simulink model "Model"  (R2024a)
settings: Solver=FixedStepDiscrete  StartTime=0.0  StopTime=inf  FixedStep=0.001  RelTol=1e-3
model workspace (MATLAB code in the model file):
  | Amplitude = 0.35/2;
settings Model: Creator=Are-Laptop  LastModifiedBy=Are-Laptop

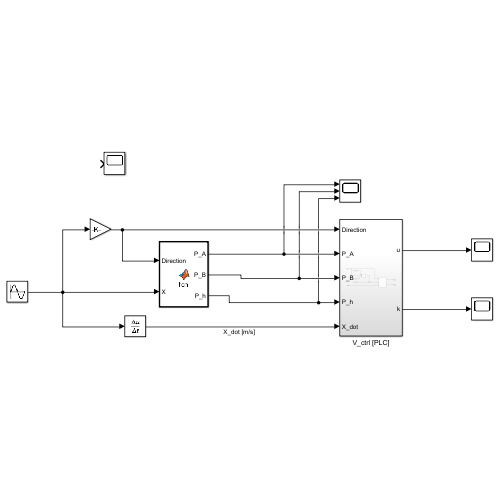
[thumbnail: Simulink's stored preview of the top-level diagram]
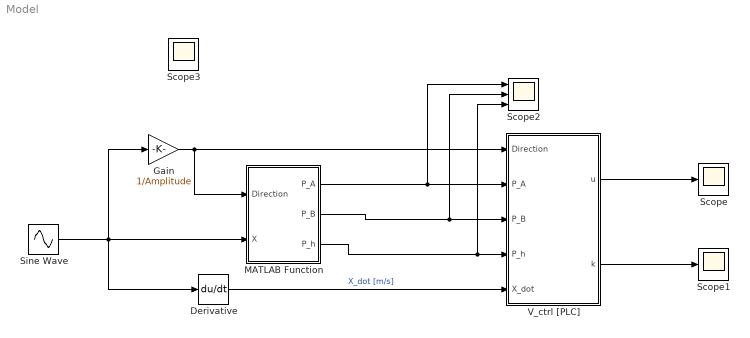
== system Model ==
  Derivative : Derivative
  Gain : Gain  Gain=1/Amplitude
  MATLAB Function : MATLAB Function  TreatAsAtomicUnit=on
  Scope : Scope
  Scope1 : Scope
  Scope2 : Scope  NumInputPorts=3
  Scope3 : Scope
  Sine Wave : Sin  Amplitude=Amplitude  Frequency=1/10  SampleTime=0
  V_ctrl [PLC] : Subsystem
  wires:
  MATLAB Function/2(P_B) -> Scope2/2, V_ctrl [PLC]/3(P_B)
  MATLAB Function/1(P_A) -> Scope2/1, V_ctrl [PLC]/2(P_A)
  MATLAB Function/3(P_h) -> Scope2/3, V_ctrl [PLC]/4(P_h)
  Derivative/1 -> V_ctrl [PLC]/5(X_dot)  "X_dot [m/s]"
  Gain/1 -> MATLAB Function/1(Direction), V_ctrl [PLC]/1(Direction)
  V_ctrl [PLC]/1(u) -> Scope/1
  V_ctrl [PLC]/2(k) -> Scope1/1
  Sine Wave/1 -> Derivative/1, Gain/1, MATLAB Function/2(X)

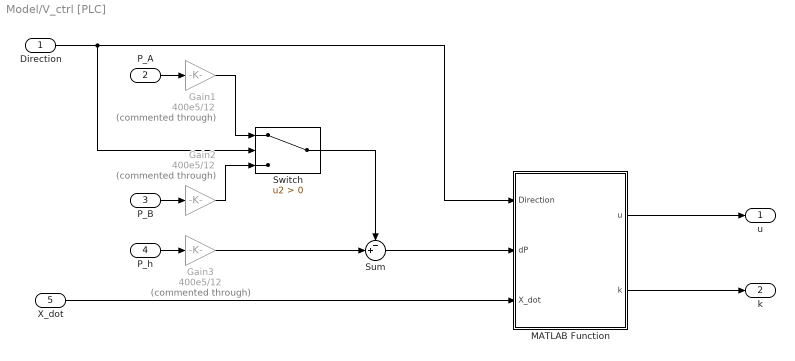
== system Model/V_ctrl [PLC] ==
  Direction : Inport
  P_A : Inport  Port=2
  P_B : Inport  Port=3
  P_h : Inport  Port=4
  X_dot : Inport  Port=5
  Gain1 : Gain  Commented=through  Gain=400e5/12
  Gain2 : Gain  Commented=through  Gain=400e5/12
  Gain3 : Gain  Commented=through  Gain=400e5/12
  MATLAB Function : MATLAB Function  TreatAsAtomicUnit=on
  Sum : Sum  Inputs=-+|
  Switch : Switch  Criteria=u2 > Threshold  SaturateOnIntegerOverflow=off  InputSameDT=off
  u : Outport
  k : Outport  Port=2
  wires:
  P_A/1 -> Gain1/1
  P_B/1 -> Gain2/1
  Direction/1 -> Switch/2, MATLAB Function/1(Direction)
  Sum/1 -> MATLAB Function/2(dP)
  P_h/1 -> Gain3/1
  Switch/1 -> Sum/1
  MATLAB Function/1(u) -> u/1
  Gain2/1 -> Switch/3
  Gain1/1 -> Switch/1
  Gain3/1 -> Sum/2
  X_dot/1 -> MATLAB Function/3(X_dot)
  MATLAB Function/2(k) -> k/1

== matlab function Model/MATLAB Function ==
  data: Direction input; P_A output; P_B output; X input; P_h output
function [P_A, P_B, P_h] = fcn(Direction, X)

%% fyske_parametere.m
% Constants
L1 = 3.625;
L4 = 0.229;
Lg4x = L1-L4/2;
Lg4y = 0.08157;
abx = 0.550;
aby = -0.130;
g = 9.81;
G1 =100*g;
G4 = (4*76+16)*g;
Cy = -1.055;
Cx = 0.420;
ang_CA = atan2(Cy,Cx);
ang_k = atan2(aby,abx);
b = abs(sqrt(Cy^2+Cx^2));
c = abs(sqrt(abx^2+aby^2));
% Calculations
%syms Ax Ay P gamma beta ang_C ang_AB r_cb r_ab L3 w_A w_C VBx VBy Vp crs_abp
L3 = X + (772+175)/1000;

ang_C = acos((L3^2+b^2-c^2)/(2*L3*b));
beta = ang_CA + pi - ang_C;

bx = L3*cos(beta) + Cx;
by = L3*sin(beta) + Cy;
ang_AB =atan2(by,bx);
gamma = ang_AB + ang_k;

r_cb = [L3*cos(beta);L3*sin(beta);0];
r_ab = [abx*cos(gamma) - aby*sin(gamma); aby*cos(gamma) + abx*sin(gamma); 0 ];
rot_rab = [-1*r_ab(2); r_ab(1)];
rot_rcb = [-1*r_cb(2); r_cb(1)];

crs_abp = cross(r_ab, [cos(beta); sin(beta);0]);
matrix = [1, 0, cos(beta);
    0, 1, sin(beta);
    0, 0, r_ab(1)*sin(beta) - r_ab(2)*cos(beta)];
right = [0;(G1+G4);(G1*cos(gamma)*L1/2+G4*(cos(gamma)*Lg4x-sin(gamma)*Lg4y))];

ANS = inv(matrix)*right;
Ax = ANS(1);
Ay = ANS(2);
P  = ANS(3);

%% pessure_compansetet.m
roh = 850;
u_0 = 0.8/7;
Ffr = 0.05*P;
A = 33.1/100^2;
A2 = 23.6/100^2;
phi = A2/A;
dp0 = 7*10^5;
Pcr = 210*10^5;
Cd = 0.6;

if Direction > 0
    % out stroke
    dp_chk = 4*10^5;
    P3 = dp0;
    P2 = (P/A + phi*P3 + Ffr/A) ;
    P1 = (P2 + dp_chk);

elseif Direction < 0
    % in stroke
    P1 = dp0;
    alpha = 3;
    M =[A, -phi*A;
        1, alpha];
    N =[P-Ffr;
        Pcr+(1+alpha)*P1];
    X = M\N;
    P2 = X(1);
    P3 = X(2);
else
    P1 = 0;
    P3 = 0;
end

P_A = P1;
P_B = P3;
P_h = 180e5;

end

== matlab function Model/V_ctrl [PLC]/MATLAB Function ==
  data: Direction input; dP input; u output; X_dot input; k output
function [u,k] = fcn(Direction, dP, X_dot)

phi = 0.7130;
A = 33.1/100^2; % Area
BW = 0.8; % Bandwidth
SpoolTravel = 7; % Maximum Spool Travel
a = (SpoolTravel-BW)/25; % Valve Slope Characteristic [mm/(L/min)]

if Direction > 0

    Q = X_dot * A; % Wanted Flow

elseif Direction < 0

    Q = X_dot * (A*phi); % Wanted Flow

else

    Q = 0; % Wanted Flow

end

dP_0 = 7e5; % Pressure drop with compansator
Q_dot = (Q * sqrt(dP_0/dP)) * 6e4; % Referance Flow [L/min]  

u = (Q_dot * a + BW)/SpoolTravel; % Control Signal [-1, 1]
k = Q * 6e4;

end
